simulink model "SimulinkTP4"  (R2018b)
settings: Solver=VariableStepAuto  StartTime=0.0  StopTime=1.5  MaxStep=1e-6  RelTol=1e-3
libraries: fl_lib x18, nesl_utility x8, elec_lib x1
settings Model: Creator=A47521  LastModifiedBy=A47521

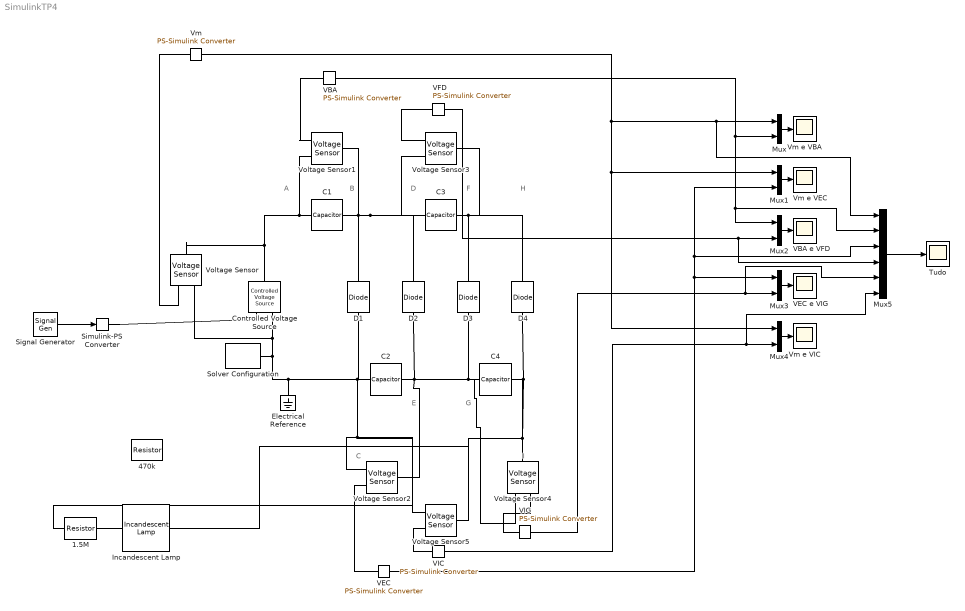
== system SimulinkTP4 ==
  note: A
  note: E
  note: F
  note: D
  note: C
  note: B
  note: G
  note: I
  note: H
  1.5M : fl_lib/Electrical/Electrical Elements/Resistor  R=1.5 MOhm  i_specify=off  i_priority=None  i=0 A  i_nominal_specify=off  i_nominal_unit=A  i_nominal_value=1  v_specify=off  v_priority=None  v=0 V  v_nominal_specify=off  v_nominal_unit=V  v_nominal_value=1
  470k : fl_lib/Electrical/Electrical Elements/Resistor  R=470 kOhm  i_specify=off  i_priority=None  i=0 A  i_nominal_specify=off  i_nominal_unit=A  i_nominal_value=1  v_specify=off  v_priority=None  v=0 V  v_nominal_specify=off  v_nominal_unit=V  v_nominal_value=1
  C{1..4} (4 alike) : fl_lib/Electrical/Electrical Elements/Capacitor  c=1 uF  r=1e-6 Ohm  g=0 1/Ohm  i_specify=off  i_priority=None  i=0 A  i_nominal_specify=off  i_nominal_unit=A  i_nominal_value=1  v_specify=off  v_priority=None  v=0 V  v_nominal_specify=off  v_nominal_unit=V  v_nominal_value=1  vc_specify=off  vc_priority=High  vc=0 V  vc_nominal_specify=off  vc_nominal_unit=V  vc_nominal_value=1
  Controlled Voltage Source : fl_lib/Electrical/Electrical Sources/Controlled Voltage Source
  D{1..4} (4 alike) : fl_lib/Electrical/Electrical Elements/Diode  Vf=0.6 V  Ron=0.3 Ohm  Goff=1e-8 1/Ohm  i_specify=off  i_priority=None  i=0 A  i_nominal_specify=off  i_nominal_unit=A  i_nominal_value=1  v_specify=off  v_priority=None  v=0 V  v_nominal_specify=off  v_nominal_unit=V  v_nominal_value=1
  Electrical Reference : fl_lib/Electrical/Electrical Elements/Electrical Reference
  Incandescent Lamp : elec_lib/Passive Devices/Incandescent Lamp  R_param=1  R0=0.15 Ohm  R1=1 Ohm  i0=70 A  i1=10 A  Vrated=24*sqrt(2) V  alpha=0.004 1/K  tc=25 ms  initial_state=1  t_fault=inf s  R_fault=1e6 Ohm
      settings: SourceProductName=Simscape Electronics  SourceProductBaseCode=SN
  Mux{,1..4} (5 alike) : Mux  Inputs=2
  Mux5 : Mux  Inputs=6
  Signal Generator : SignalGenerator  Amplitude=24*sqrt(2)  Frequency=50
  Simulink-PS Converter : nesl_utility/Simulink-PS Converter  PhysicalDomain=network_engine_domain  SubClassName=ps_input  LeftPortType=input  RightPortType=output  PseudoPeriodic=off  Frequencies=[]  NoiseDistribution=none  NoiseParameters=[]  Unit=1  AffineConversion=off  FilteringAndDerivatives=provide  SimscapeFilterOrder=1  InputFilterTimeConstant=0.001  UdotUserProvided=0
  Solver Configuration : nesl_utility/Solver Configuration  PhysicalDomain=network_engine_domain  SubClassName=solver  LeftPortType=input  RightPortType=generic  Tones=[]  Harmonics=[]  SimulateNoise=off  Profile=off  UseLocalSampling=off  EnableSwitchedLinearOptims=on  FrequencyDomain=off  UseCCode=off  RelTol=0.001  AbsTol=1e-06  MinStep=1e-09  ToWorkspace=off  RevertToSquareIcSolve=off  NumHomotopyIterations=100  PhasorMode=off  PhasorModeNumHarmonics=1  DoDC=off  ResidualTolerance=1e-09  UseLocalSolver=off  LocalSolverChoice=NE_BACKWARD_EULER_ADVANCER  LocalSolverSampleTime=0.001  DoFixedCost=off  MaxNonlinIter=3  MaxModeIter=2  LinearAlgebra=auto  EquationFormulation=NE_TIME_EF  DelaysMemoryBudget=1024  AutomaticFiltering=on  FilteringTimeConstant=0.001  PartitionStorageMethod=AS_NEEDED  PartitionMemoryBudget=1024
  Tudo : Scope
  VBA : nesl_utility/PS-Simulink Converter  PhysicalDomain=network_engine_domain  SubClassName=ps_output  LeftPortType=input  RightPortType=output  PseudoPeriodic=off  Frequencies=[]  Unit=1  AffineConversion=off
  VBA e VFD : Scope
  VEC : nesl_utility/PS-Simulink Converter  PhysicalDomain=network_engine_domain  SubClassName=ps_output  LeftPortType=input  RightPortType=output  PseudoPeriodic=off  Frequencies=[]  Unit=1  AffineConversion=off
  VEC e VIG : Scope
  VFD : nesl_utility/PS-Simulink Converter  PhysicalDomain=network_engine_domain  SubClassName=ps_output  LeftPortType=input  RightPortType=output  PseudoPeriodic=off  Frequencies=[]  Unit=1  AffineConversion=off
  VIC : nesl_utility/PS-Simulink Converter  PhysicalDomain=network_engine_domain  SubClassName=ps_output  LeftPortType=input  RightPortType=output  PseudoPeriodic=off  Frequencies=[]  Unit=1  AffineConversion=off
  VIG : nesl_utility/PS-Simulink Converter  PhysicalDomain=network_engine_domain  SubClassName=ps_output  LeftPortType=input  RightPortType=output  PseudoPeriodic=off  Frequencies=[]  Unit=1  AffineConversion=off
  Vm : nesl_utility/PS-Simulink Converter  PhysicalDomain=network_engine_domain  SubClassName=ps_output  LeftPortType=input  RightPortType=output  PseudoPeriodic=off  Frequencies=[]  Unit=1  AffineConversion=off
  Vm e VBA : Scope
  Vm e VEC : Scope
  Vm e VIC : Scope
  Voltage Sensor{,1..5} (6 alike) : fl_lib/Electrical/Electrical Sensors/Voltage Sensor
  wires:
  Signal Generator/1 -> Simulink-PS Converter/1
  Mux/1 -> Vm e VBA/1
  Mux1/1 -> Vm e VEC/1
  Mux2/1 -> VBA e VFD/1
  Mux3/1 -> VEC e VIG/1
  Mux4/1 -> Vm e VIC/1
  Vm/1 -> Mux1/1, Mux4/1, Mux5/1, Mux/1
  VEC/1 -> Mux5/3, Mux1/2, Mux3/1
  VIG/1 -> Mux5/5, Mux3/2
  VBA/1 -> Mux/2, Mux5/2, Mux2/1
  VFD/1 -> Mux5/4, Mux2/2
  Mux5/1 -> Tudo/1
  VIC/1 -> Mux5/6, Mux4/2
  connections:
  Simulink-PS Converter/RConn1 -- Controlled Voltage Source/RConn1
  Controlled Voltage Source/RConn2 -- Voltage Sensor/RConn2 -- Electrical Reference/LConn1 -- D1/LConn1 -- C2/RConn1 -- 1.5M/LConn1 -- Voltage Sensor5/RConn2 -- Voltage Sensor2/RConn2 -- Solver Configuration/RConn1
  Controlled Voltage Source/LConn1 -- Voltage Sensor/LConn1 -- Voltage Sensor1/RConn2 -- C1/RConn1
  C2/LConn1 -- Voltage Sensor2/LConn1 -- Voltage Sensor4/RConn2 -- D3/LConn1 -- C4/RConn1 -- D2/RConn1
  C1/LConn1 -- D2/LConn1 -- C3/RConn1 -- Voltage Sensor3/RConn2 -- Voltage Sensor1/LConn1 -- D1/RConn1
  D3/RConn1 -- Voltage Sensor3/LConn1 -- D4/LConn1 -- C3/LConn1
  C4/LConn1 -- Incandescent Lamp/RConn1 -- Voltage Sensor5/LConn1 -- Voltage Sensor4/LConn1 -- D4/RConn1
  Voltage Sensor/RConn1 -- Vm/LConn1
  Voltage Sensor1/RConn1 -- VBA/LConn1
  Voltage Sensor3/RConn1 -- VFD/LConn1
  VIG/LConn1 -- Voltage Sensor4/RConn1
  Voltage Sensor5/RConn1 -- VIC/LConn1
  Voltage Sensor2/RConn1 -- VEC/LConn1
  1.5M/RConn1 -- Incandescent Lamp/LConn1
